simulink model "rx2"  (R2022b)
settings: Solver=FixedStepDiscrete  StartTime=0.0  StopTime=3.3E6  FixedStep=1  RelTol=1e-3  EnableMultiTasking=on
model workspace (MAT data in the model file):
  mwTaskManagerKernelLatency = 0
undefined symbols (not defined in the file or in its folder): Add, jsin, magnitude, rom_pilot_conj_tt, Shift
libraries: hdlsllib x3231, whdlutilities x525, simulink x260, whdlmod x112, whdledac x26, dsphdlmathfun2 x24, commchan3 x1
(part 42 of 59)

== system rx2/process3/decoder/p-p/Subsystem2/Subsystem1 ==
  data1 : Inport  OutDataTypeStr=data_type
  wr_addr : Inport  Port=2
  wr_en1 : Inport  Port=3
  rd_addr : Inport  Port=4
  Mux : Mux  Inputs=2
  Selector : Selector  InputPortWidth=32  IndexOptions=Index vector (dialog)  Indices=[1:16]  OutputSizes=1
  Selector1 : Selector  InputPortWidth=32  IndexOptions=Index vector (dialog)  Indices=[17:32]  OutputSizes=1
  Subsystem1 : Subsystem
  Subsystem2 : Subsystem
  rd_dout : Outport  PortDimensions=32  VectorParamsAs1DForOutWhenUnconnected=off
  wires:
  Selector1/1 -> Subsystem1/1(data1)
  Selector/1 -> Subsystem2/1(data1)
  rd_addr/1 -> Subsystem2/4(rd_addr), Subsystem1/4(rd_addr)
  Mux/1 -> rd_dout/1
  wr_en1/1 -> Subsystem2/3(wr_en1), Subsystem1/3(wr_en1)
  Subsystem2/1(rd_dout) -> Mux/1
  Subsystem1/1(rd_dout) -> Mux/2
  wr_addr/1 -> Subsystem2/2(wr_addr), Subsystem1/2(wr_addr)
  data1/1 -> Selector1/1, Selector/1

== system rx2/process3/decoder/p-p/p_s_new/Subsystem1 ==
  In1 : Inport
  Demux{,1..6} (7 alike) : Demux  Outputs=2
  Out1 : Outport
  Out2 : Outport  Port=2
  Out3 : Outport  Port=3
  Out4 : Outport  Port=4
  Out5 : Outport  Port=5
  Out6 : Outport  Port=6
  Out7 : Outport  Port=7
  Out8 : Outport  Port=8
  wires:
  Demux3/1 -> Out1/1
  Demux6/2 -> Out8/1
  Demux4/2 -> Out4/1
  Demux5/1 -> Out5/1
  In1/1 -> Demux2/1
  Demux5/2 -> Out6/1
  Demux3/2 -> Out2/1
  Demux1/1 -> Demux5/1
  Demux/2 -> Demux4/1
  Demux1/2 -> Demux6/1
  Demux6/1 -> Out7/1
  Demux2/2 -> Demux1/1
  Demux/1 -> Demux3/1
  Demux4/1 -> Out3/1
  Demux2/1 -> Demux/1

== system rx2/process3/decoder/p-p/p_s_new/Subsystem3 ==
  In1 : Inport
  Demux{,1..6} (7 alike) : Demux  Outputs=2
  Out1 : Outport
  Out2 : Outport  Port=2
  Out3 : Outport  Port=3
  Out4 : Outport  Port=4
  Out5 : Outport  Port=5
  Out6 : Outport  Port=6
  Out7 : Outport  Port=7
  Out8 : Outport  Port=8
  wires:
  Demux2/1 -> Demux/1
  Demux4/1 -> Out3/1
  Demux/1 -> Demux3/1
  Demux2/2 -> Demux1/1
  Demux6/1 -> Out7/1
  Demux1/2 -> Demux6/1
  Demux/2 -> Demux4/1
  Demux1/1 -> Demux5/1
  Demux3/2 -> Out2/1
  Demux5/2 -> Out6/1
  In1/1 -> Demux2/1
  Demux5/1 -> Out5/1
  Demux4/2 -> Out4/1
  Demux6/2 -> Out8/1
  Demux3/1 -> Out1/1

== system rx2/process3/decoder/p-p/p_s_new/Subsystem4 ==
  In1 : Inport
  Demux{,1..6} (7 alike) : Demux  Outputs=2
  Out1 : Outport
  Out2 : Outport  Port=2
  Out3 : Outport  Port=3
  Out4 : Outport  Port=4
  Out5 : Outport  Port=5
  Out6 : Outport  Port=6
  Out7 : Outport  Port=7
  Out8 : Outport  Port=8
  wires:
  Demux3/1 -> Out1/1
  Demux6/2 -> Out8/1
  Demux4/2 -> Out4/1
  Demux5/1 -> Out5/1
  In1/1 -> Demux2/1
  Demux5/2 -> Out6/1
  Demux3/2 -> Out2/1
  Demux1/1 -> Demux5/1
  Demux/2 -> Demux4/1
  Demux1/2 -> Demux6/1
  Demux6/1 -> Out7/1
  Demux2/2 -> Demux1/1
  Demux/1 -> Demux3/1
  Demux4/1 -> Out3/1
  Demux2/1 -> Demux/1

== system rx2/process3/decoder/p-p/p_s_new/Subsystem5 ==
  In1 : Inport
  Demux{,1..6} (7 alike) : Demux  Outputs=2
  Out1 : Outport
  Out2 : Outport  Port=2
  Out3 : Outport  Port=3
  Out4 : Outport  Port=4
  Out5 : Outport  Port=5
  Out6 : Outport  Port=6
  Out7 : Outport  Port=7
  Out8 : Outport  Port=8
  wires:
  Demux2/1 -> Demux/1
  Demux4/1 -> Out3/1
  Demux/1 -> Demux3/1
  Demux2/2 -> Demux1/1
  Demux6/1 -> Out7/1
  Demux1/2 -> Demux6/1
  Demux/2 -> Demux4/1
  Demux1/1 -> Demux5/1
  Demux3/2 -> Out2/1
  Demux5/2 -> Out6/1
  In1/1 -> Demux2/1
  Demux5/1 -> Out5/1
  Demux4/2 -> Out4/1
  Demux6/2 -> Out8/1
  Demux3/1 -> Out1/1

== system rx2/process4/decoder/p-p/Subsystem2/Subsystem ==
  data1 : Inport  OutDataTypeStr=data_type
  wr_addr : Inport  Port=2
  wr_en1 : Inport  Port=3
  rd_addr : Inport  Port=4
  Mux : Mux  Inputs=2
  Selector : Selector  InputPortWidth=32  IndexOptions=Index vector (dialog)  Indices=[1:16]  OutputSizes=1
  Selector1 : Selector  InputPortWidth=32  IndexOptions=Index vector (dialog)  Indices=[17:32]  OutputSizes=1
  Subsystem1 : Subsystem
  Subsystem2 : Subsystem
  rd_dout : Outport  PortDimensions=32  VectorParamsAs1DForOutWhenUnconnected=off
  wires:
  data1/1 -> Selector/1, Selector1/1
  wr_addr/1 -> Subsystem1/2(wr_addr), Subsystem2/2(wr_addr)
  Subsystem1/1(rd_dout) -> Mux/2
  Subsystem2/1(rd_dout) -> Mux/1
  wr_en1/1 -> Subsystem1/3(wr_en1), Subsystem2/3(wr_en1)
  Mux/1 -> rd_dout/1
  rd_addr/1 -> Subsystem1/4(rd_addr), Subsystem2/4(rd_addr)
  Selector/1 -> Subsystem2/1(data1)
  Selector1/1 -> Subsystem1/1(data1)

== system rx2/process4/decoder/p-p/Subsystem2/Subsystem1 ==
  data1 : Inport  OutDataTypeStr=data_type
  wr_addr : Inport  Port=2
  wr_en1 : Inport  Port=3
  rd_addr : Inport  Port=4
  Mux : Mux  Inputs=2
  Selector : Selector  InputPortWidth=32  IndexOptions=Index vector (dialog)  Indices=[1:16]  OutputSizes=1
  Selector1 : Selector  InputPortWidth=32  IndexOptions=Index vector (dialog)  Indices=[17:32]  OutputSizes=1
  Subsystem1 : Subsystem
  Subsystem2 : Subsystem
  rd_dout : Outport  PortDimensions=32  VectorParamsAs1DForOutWhenUnconnected=off
  wires:
  data1/1 -> Selector/1, Selector1/1
  wr_addr/1 -> Subsystem1/2(wr_addr), Subsystem2/2(wr_addr)
  Subsystem1/1(rd_dout) -> Mux/2
  Subsystem2/1(rd_dout) -> Mux/1
  wr_en1/1 -> Subsystem1/3(wr_en1), Subsystem2/3(wr_en1)
  Mux/1 -> rd_dout/1
  rd_addr/1 -> Subsystem1/4(rd_addr), Subsystem2/4(rd_addr)
  Selector/1 -> Subsystem2/1(data1)
  Selector1/1 -> Subsystem1/1(data1)

== system rx2/process4/decoder/p-p/p_s_new/Subsystem1 ==
  In1 : Inport
  Demux{,1..6} (7 alike) : Demux  Outputs=2
  Out1 : Outport
  Out2 : Outport  Port=2
  Out3 : Outport  Port=3
  Out4 : Outport  Port=4
  Out5 : Outport  Port=5
  Out6 : Outport  Port=6
  Out7 : Outport  Port=7
  Out8 : Outport  Port=8
  wires:
  Demux2/1 -> Demux/1
  Demux4/1 -> Out3/1
  Demux/1 -> Demux3/1
  Demux2/2 -> Demux1/1
  Demux6/1 -> Out7/1
  Demux1/2 -> Demux6/1
  Demux/2 -> Demux4/1
  Demux1/1 -> Demux5/1
  Demux3/2 -> Out2/1
  Demux5/2 -> Out6/1
  In1/1 -> Demux2/1
  Demux5/1 -> Out5/1
  Demux4/2 -> Out4/1
  Demux6/2 -> Out8/1
  Demux3/1 -> Out1/1

== system rx2/process4/decoder/p-p/p_s_new/Subsystem3 ==
  In1 : Inport
  Demux{,1..6} (7 alike) : Demux  Outputs=2
  Out1 : Outport
  Out2 : Outport  Port=2
  Out3 : Outport  Port=3
  Out4 : Outport  Port=4
  Out5 : Outport  Port=5
  Out6 : Outport  Port=6
  Out7 : Outport  Port=7
  Out8 : Outport  Port=8
  wires:
  Demux3/1 -> Out1/1
  Demux6/2 -> Out8/1
  Demux4/2 -> Out4/1
  Demux5/1 -> Out5/1
  In1/1 -> Demux2/1
  Demux5/2 -> Out6/1
  Demux3/2 -> Out2/1
  Demux1/1 -> Demux5/1
  Demux/2 -> Demux4/1
  Demux1/2 -> Demux6/1
  Demux6/1 -> Out7/1
  Demux2/2 -> Demux1/1
  Demux/1 -> Demux3/1
  Demux4/1 -> Out3/1
  Demux2/1 -> Demux/1

== system rx2/process4/decoder/p-p/p_s_new/Subsystem4 ==
  In1 : Inport
  Demux{,1..6} (7 alike) : Demux  Outputs=2
  Out1 : Outport
  Out2 : Outport  Port=2
  Out3 : Outport  Port=3
  Out4 : Outport  Port=4
  Out5 : Outport  Port=5
  Out6 : Outport  Port=6
  Out7 : Outport  Port=7
  Out8 : Outport  Port=8
  wires:
  Demux2/1 -> Demux/1
  Demux4/1 -> Out3/1
  Demux/1 -> Demux3/1
  Demux2/2 -> Demux1/1
  Demux6/1 -> Out7/1
  Demux1/2 -> Demux6/1
  Demux/2 -> Demux4/1
  Demux1/1 -> Demux5/1
  Demux3/2 -> Out2/1
  Demux5/2 -> Out6/1
  In1/1 -> Demux2/1
  Demux5/1 -> Out5/1
  Demux4/2 -> Out4/1
  Demux6/2 -> Out8/1
  Demux3/1 -> Out1/1

== system rx2/process4/decoder/p-p/p_s_new/Subsystem5 ==
  In1 : Inport
  Demux{,1..6} (7 alike) : Demux  Outputs=2
  Out1 : Outport
  Out2 : Outport  Port=2
  Out3 : Outport  Port=3
  Out4 : Outport  Port=4
  Out5 : Outport  Port=5
  Out6 : Outport  Port=6
  Out7 : Outport  Port=7
  Out8 : Outport  Port=8
  wires:
  Demux3/1 -> Out1/1
  Demux6/2 -> Out8/1
  Demux4/2 -> Out4/1
  Demux5/1 -> Out5/1
  In1/1 -> Demux2/1
  Demux5/2 -> Out6/1
  Demux3/2 -> Out2/1
  Demux1/1 -> Demux5/1
  Demux/2 -> Demux4/1
  Demux1/2 -> Demux6/1
  Demux6/1 -> Out7/1
  Demux2/2 -> Demux1/1
  Demux/1 -> Demux3/1
  Demux4/1 -> Out3/1
  Demux2/1 -> Demux/1

== system rx2/process5/decoder/p-p/Subsystem2/Subsystem ==
  data1 : Inport  OutDataTypeStr=data_type
  wr_addr : Inport  Port=2
  wr_en1 : Inport  Port=3
  rd_addr : Inport  Port=4
  Mux : Mux  Inputs=2
  Selector : Selector  InputPortWidth=32  IndexOptions=Index vector (dialog)  Indices=[1:16]  OutputSizes=1
  Selector1 : Selector  InputPortWidth=32  IndexOptions=Index vector (dialog)  Indices=[17:32]  OutputSizes=1
  Subsystem1 : Subsystem
  Subsystem2 : Subsystem
  rd_dout : Outport  PortDimensions=32  VectorParamsAs1DForOutWhenUnconnected=off
  wires:
  Selector1/1 -> Subsystem1/1(data1)
  Selector/1 -> Subsystem2/1(data1)
  rd_addr/1 -> Subsystem2/4(rd_addr), Subsystem1/4(rd_addr)
  Mux/1 -> rd_dout/1
  wr_en1/1 -> Subsystem2/3(wr_en1), Subsystem1/3(wr_en1)
  Subsystem2/1(rd_dout) -> Mux/1
  Subsystem1/1(rd_dout) -> Mux/2
  wr_addr/1 -> Subsystem2/2(wr_addr), Subsystem1/2(wr_addr)
  data1/1 -> Selector1/1, Selector/1

== system rx2/process5/decoder/p-p/Subsystem2/Subsystem1 ==
  data1 : Inport  OutDataTypeStr=data_type
  wr_addr : Inport  Port=2
  wr_en1 : Inport  Port=3
  rd_addr : Inport  Port=4
  Mux : Mux  Inputs=2
  Selector : Selector  InputPortWidth=32  IndexOptions=Index vector (dialog)  Indices=[1:16]  OutputSizes=1
  Selector1 : Selector  InputPortWidth=32  IndexOptions=Index vector (dialog)  Indices=[17:32]  OutputSizes=1
  Subsystem1 : Subsystem
  Subsystem2 : Subsystem
  rd_dout : Outport  PortDimensions=32  VectorParamsAs1DForOutWhenUnconnected=off
  wires:
  Selector1/1 -> Subsystem1/1(data1)
  Selector/1 -> Subsystem2/1(data1)
  rd_addr/1 -> Subsystem2/4(rd_addr), Subsystem1/4(rd_addr)
  Mux/1 -> rd_dout/1
  wr_en1/1 -> Subsystem2/3(wr_en1), Subsystem1/3(wr_en1)
  Subsystem2/1(rd_dout) -> Mux/1
  Subsystem1/1(rd_dout) -> Mux/2
  wr_addr/1 -> Subsystem2/2(wr_addr), Subsystem1/2(wr_addr)
  data1/1 -> Selector1/1, Selector/1

== system rx2/process5/decoder/p-p/p_s_new/Subsystem1 ==
  In1 : Inport
  Demux{,1..6} (7 alike) : Demux  Outputs=2
  Out1 : Outport
  Out2 : Outport  Port=2
  Out3 : Outport  Port=3
  Out4 : Outport  Port=4
  Out5 : Outport  Port=5
  Out6 : Outport  Port=6
  Out7 : Outport  Port=7
  Out8 : Outport  Port=8
  wires:
  Demux3/1 -> Out1/1
  Demux6/2 -> Out8/1
  Demux4/2 -> Out4/1
  Demux5/1 -> Out5/1
  In1/1 -> Demux2/1
  Demux5/2 -> Out6/1
  Demux3/2 -> Out2/1
  Demux1/1 -> Demux5/1
  Demux/2 -> Demux4/1
  Demux1/2 -> Demux6/1
  Demux6/1 -> Out7/1
  Demux2/2 -> Demux1/1
  Demux/1 -> Demux3/1
  Demux4/1 -> Out3/1
  Demux2/1 -> Demux/1

== system rx2/process5/decoder/p-p/p_s_new/Subsystem3 ==
  In1 : Inport
  Demux{,1..6} (7 alike) : Demux  Outputs=2
  Out1 : Outport
  Out2 : Outport  Port=2
  Out3 : Outport  Port=3
  Out4 : Outport  Port=4
  Out5 : Outport  Port=5
  Out6 : Outport  Port=6
  Out7 : Outport  Port=7
  Out8 : Outport  Port=8
  wires:
  Demux2/1 -> Demux/1
  Demux4/1 -> Out3/1
  Demux/1 -> Demux3/1
  Demux2/2 -> Demux1/1
  Demux6/1 -> Out7/1
  Demux1/2 -> Demux6/1
  Demux/2 -> Demux4/1
  Demux1/1 -> Demux5/1
  Demux3/2 -> Out2/1
  Demux5/2 -> Out6/1
  In1/1 -> Demux2/1
  Demux5/1 -> Out5/1
  Demux4/2 -> Out4/1
  Demux6/2 -> Out8/1
  Demux3/1 -> Out1/1

== system rx2/process5/decoder/p-p/p_s_new/Subsystem4 ==
  In1 : Inport
  Demux{,1..6} (7 alike) : Demux  Outputs=2
  Out1 : Outport
  Out2 : Outport  Port=2
  Out3 : Outport  Port=3
  Out4 : Outport  Port=4
  Out5 : Outport  Port=5
  Out6 : Outport  Port=6
  Out7 : Outport  Port=7
  Out8 : Outport  Port=8
  wires:
  Demux3/1 -> Out1/1
  Demux6/2 -> Out8/1
  Demux4/2 -> Out4/1
  Demux5/1 -> Out5/1
  In1/1 -> Demux2/1
  Demux5/2 -> Out6/1
  Demux3/2 -> Out2/1
  Demux1/1 -> Demux5/1
  Demux/2 -> Demux4/1
  Demux1/2 -> Demux6/1
  Demux6/1 -> Out7/1
  Demux2/2 -> Demux1/1
  Demux/1 -> Demux3/1
  Demux4/1 -> Out3/1
  Demux2/1 -> Demux/1

== system rx2/process5/decoder/p-p/p_s_new/Subsystem5 ==
  In1 : Inport
  Demux{,1..6} (7 alike) : Demux  Outputs=2
  Out1 : Outport
  Out2 : Outport  Port=2
  Out3 : Outport  Port=3
  Out4 : Outport  Port=4
  Out5 : Outport  Port=5
  Out6 : Outport  Port=6
  Out7 : Outport  Port=7
  Out8 : Outport  Port=8
  wires:
  Demux2/1 -> Demux/1
  Demux4/1 -> Out3/1
  Demux/1 -> Demux3/1
  Demux2/2 -> Demux1/1
  Demux6/1 -> Out7/1
  Demux1/2 -> Demux6/1
  Demux/2 -> Demux4/1
  Demux1/1 -> Demux5/1
  Demux3/2 -> Out2/1
  Demux5/2 -> Out6/1
  In1/1 -> Demux2/1
  Demux5/1 -> Out5/1
  Demux4/2 -> Out4/1
  Demux6/2 -> Out8/1
  Demux3/1 -> Out1/1

== system rx2/process6/decoder/p-p/Subsystem2/Subsystem ==
  data1 : Inport  OutDataTypeStr=data_type
  wr_addr : Inport  Port=2
  wr_en1 : Inport  Port=3
  rd_addr : Inport  Port=4
  Mux : Mux  Inputs=2
  Selector : Selector  InputPortWidth=32  IndexOptions=Index vector (dialog)  Indices=[1:16]  OutputSizes=1
  Selector1 : Selector  InputPortWidth=32  IndexOptions=Index vector (dialog)  Indices=[17:32]  OutputSizes=1
  Subsystem1 : Subsystem
  Subsystem2 : Subsystem
  rd_dout : Outport  PortDimensions=32  VectorParamsAs1DForOutWhenUnconnected=off
  wires:
  data1/1 -> Selector/1, Selector1/1
  wr_addr/1 -> Subsystem1/2(wr_addr), Subsystem2/2(wr_addr)
  Subsystem1/1(rd_dout) -> Mux/2
  Subsystem2/1(rd_dout) -> Mux/1
  wr_en1/1 -> Subsystem1/3(wr_en1), Subsystem2/3(wr_en1)
  Mux/1 -> rd_dout/1
  rd_addr/1 -> Subsystem1/4(rd_addr), Subsystem2/4(rd_addr)
  Selector/1 -> Subsystem2/1(data1)
  Selector1/1 -> Subsystem1/1(data1)

== system rx2/process6/decoder/p-p/Subsystem2/Subsystem1 ==
  data1 : Inport  OutDataTypeStr=data_type
  wr_addr : Inport  Port=2
  wr_en1 : Inport  Port=3
  rd_addr : Inport  Port=4
  Mux : Mux  Inputs=2
  Selector : Selector  InputPortWidth=32  IndexOptions=Index vector (dialog)  Indices=[1:16]  OutputSizes=1
  Selector1 : Selector  InputPortWidth=32  IndexOptions=Index vector (dialog)  Indices=[17:32]  OutputSizes=1
  Subsystem1 : Subsystem
  Subsystem2 : Subsystem
  rd_dout : Outport  PortDimensions=32  VectorParamsAs1DForOutWhenUnconnected=off
  wires:
  data1/1 -> Selector/1, Selector1/1
  wr_addr/1 -> Subsystem1/2(wr_addr), Subsystem2/2(wr_addr)
  Subsystem1/1(rd_dout) -> Mux/2
  Subsystem2/1(rd_dout) -> Mux/1
  wr_en1/1 -> Subsystem1/3(wr_en1), Subsystem2/3(wr_en1)
  Mux/1 -> rd_dout/1
  rd_addr/1 -> Subsystem1/4(rd_addr), Subsystem2/4(rd_addr)
  Selector/1 -> Subsystem2/1(data1)
  Selector1/1 -> Subsystem1/1(data1)

== system rx2/process6/decoder/p-p/p_s_new/Subsystem1 ==
  In1 : Inport
  Demux{,1..6} (7 alike) : Demux  Outputs=2
  Out1 : Outport
  Out2 : Outport  Port=2
  Out3 : Outport  Port=3
  Out4 : Outport  Port=4
  Out5 : Outport  Port=5
  Out6 : Outport  Port=6
  Out7 : Outport  Port=7
  Out8 : Outport  Port=8
  wires:
  Demux2/1 -> Demux/1
  Demux4/1 -> Out3/1
  Demux/1 -> Demux3/1
  Demux2/2 -> Demux1/1
  Demux6/1 -> Out7/1
  Demux1/2 -> Demux6/1
  Demux/2 -> Demux4/1
  Demux1/1 -> Demux5/1
  Demux3/2 -> Out2/1
  Demux5/2 -> Out6/1
  In1/1 -> Demux2/1
  Demux5/1 -> Out5/1
  Demux4/2 -> Out4/1
  Demux6/2 -> Out8/1
  Demux3/1 -> Out1/1

== system rx2/process6/decoder/p-p/p_s_new/Subsystem3 ==
  In1 : Inport
  Demux{,1..6} (7 alike) : Demux  Outputs=2
  Out1 : Outport
  Out2 : Outport  Port=2
  Out3 : Outport  Port=3
  Out4 : Outport  Port=4
  Out5 : Outport  Port=5
  Out6 : Outport  Port=6
  Out7 : Outport  Port=7
  Out8 : Outport  Port=8
  wires:
  Demux3/1 -> Out1/1
  Demux6/2 -> Out8/1
  Demux4/2 -> Out4/1
  Demux5/1 -> Out5/1
  In1/1 -> Demux2/1
  Demux5/2 -> Out6/1
  Demux3/2 -> Out2/1
  Demux1/1 -> Demux5/1
  Demux/2 -> Demux4/1
  Demux1/2 -> Demux6/1
  Demux6/1 -> Out7/1
  Demux2/2 -> Demux1/1
  Demux/1 -> Demux3/1
  Demux4/1 -> Out3/1
  Demux2/1 -> Demux/1

== system rx2/process6/decoder/p-p/p_s_new/Subsystem4 ==
  In1 : Inport
  Demux{,1..6} (7 alike) : Demux  Outputs=2
  Out1 : Outport
  Out2 : Outport  Port=2
  Out3 : Outport  Port=3
  Out4 : Outport  Port=4
  Out5 : Outport  Port=5
  Out6 : Outport  Port=6
  Out7 : Outport  Port=7
  Out8 : Outport  Port=8
  wires:
  Demux2/1 -> Demux/1
  Demux4/1 -> Out3/1
  Demux/1 -> Demux3/1
  Demux2/2 -> Demux1/1
  Demux6/1 -> Out7/1
  Demux1/2 -> Demux6/1
  Demux/2 -> Demux4/1
  Demux1/1 -> Demux5/1
  Demux3/2 -> Out2/1
  Demux5/2 -> Out6/1
  In1/1 -> Demux2/1
  Demux5/1 -> Out5/1
  Demux4/2 -> Out4/1
  Demux6/2 -> Out8/1
  Demux3/1 -> Out1/1

== system rx2/process6/decoder/p-p/p_s_new/Subsystem5 ==
  In1 : Inport
  Demux{,1..6} (7 alike) : Demux  Outputs=2
  Out1 : Outport
  Out2 : Outport  Port=2
  Out3 : Outport  Port=3
  Out4 : Outport  Port=4
  Out5 : Outport  Port=5
  Out6 : Outport  Port=6
  Out7 : Outport  Port=7
  Out8 : Outport  Port=8
  wires:
  Demux3/1 -> Out1/1
  Demux6/2 -> Out8/1
  Demux4/2 -> Out4/1
  Demux5/1 -> Out5/1
  In1/1 -> Demux2/1
  Demux5/2 -> Out6/1
  Demux3/2 -> Out2/1
  Demux1/1 -> Demux5/1
  Demux/2 -> Demux4/1
  Demux1/2 -> Demux6/1
  Demux6/1 -> Out7/1
  Demux2/2 -> Demux1/1
  Demux/1 -> Demux3/1
  Demux4/1 -> Out3/1
  Demux2/1 -> Demux/1

== system rx2/process7/decoder/p-p/Subsystem2/Subsystem ==
  data1 : Inport  OutDataTypeStr=data_type
  wr_addr : Inport  Port=2
  wr_en1 : Inport  Port=3
  rd_addr : Inport  Port=4
  Mux : Mux  Inputs=2
  Selector : Selector  InputPortWidth=32  IndexOptions=Index vector (dialog)  Indices=[1:16]  OutputSizes=1
  Selector1 : Selector  InputPortWidth=32  IndexOptions=Index vector (dialog)  Indices=[17:32]  OutputSizes=1
  Subsystem1 : Subsystem
  Subsystem2 : Subsystem
  rd_dout : Outport  PortDimensions=32  VectorParamsAs1DForOutWhenUnconnected=off
  wires:
  Selector1/1 -> Subsystem1/1(data1)
  Selector/1 -> Subsystem2/1(data1)
  rd_addr/1 -> Subsystem2/4(rd_addr), Subsystem1/4(rd_addr)
  Mux/1 -> rd_dout/1
  wr_en1/1 -> Subsystem2/3(wr_en1), Subsystem1/3(wr_en1)
  Subsystem2/1(rd_dout) -> Mux/1
  Subsystem1/1(rd_dout) -> Mux/2
  wr_addr/1 -> Subsystem2/2(wr_addr), Subsystem1/2(wr_addr)
  data1/1 -> Selector1/1, Selector/1

== system rx2/process7/decoder/p-p/Subsystem2/Subsystem1 ==
  data1 : Inport  OutDataTypeStr=data_type
  wr_addr : Inport  Port=2
  wr_en1 : Inport  Port=3
  rd_addr : Inport  Port=4
  Mux : Mux  Inputs=2
  Selector : Selector  InputPortWidth=32  IndexOptions=Index vector (dialog)  Indices=[1:16]  OutputSizes=1
  Selector1 : Selector  InputPortWidth=32  IndexOptions=Index vector (dialog)  Indices=[17:32]  OutputSizes=1
  Subsystem1 : Subsystem
  Subsystem2 : Subsystem
  rd_dout : Outport  PortDimensions=32  VectorParamsAs1DForOutWhenUnconnected=off
  wires:
  Selector1/1 -> Subsystem1/1(data1)
  Selector/1 -> Subsystem2/1(data1)
  rd_addr/1 -> Subsystem2/4(rd_addr), Subsystem1/4(rd_addr)
  Mux/1 -> rd_dout/1
  wr_en1/1 -> Subsystem2/3(wr_en1), Subsystem1/3(wr_en1)
  Subsystem2/1(rd_dout) -> Mux/1
  Subsystem1/1(rd_dout) -> Mux/2
  wr_addr/1 -> Subsystem2/2(wr_addr), Subsystem1/2(wr_addr)
  data1/1 -> Selector1/1, Selector/1

== system rx2/process7/decoder/p-p/p_s_new/Subsystem1 ==
  In1 : Inport
  Demux{,1..6} (7 alike) : Demux  Outputs=2
  Out1 : Outport
  Out2 : Outport  Port=2
  Out3 : Outport  Port=3
  Out4 : Outport  Port=4
  Out5 : Outport  Port=5
  Out6 : Outport  Port=6
  Out7 : Outport  Port=7
  Out8 : Outport  Port=8
  wires:
  Demux3/1 -> Out1/1
  Demux6/2 -> Out8/1
  Demux4/2 -> Out4/1
  Demux5/1 -> Out5/1
  In1/1 -> Demux2/1
  Demux5/2 -> Out6/1
  Demux3/2 -> Out2/1
  Demux1/1 -> Demux5/1
  Demux/2 -> Demux4/1
  Demux1/2 -> Demux6/1
  Demux6/1 -> Out7/1
  Demux2/2 -> Demux1/1
  Demux/1 -> Demux3/1
  Demux4/1 -> Out3/1
  Demux2/1 -> Demux/1

== system rx2/process7/decoder/p-p/p_s_new/Subsystem3 ==
  In1 : Inport
  Demux{,1..6} (7 alike) : Demux  Outputs=2
  Out1 : Outport
  Out2 : Outport  Port=2
  Out3 : Outport  Port=3
  Out4 : Outport  Port=4
  Out5 : Outport  Port=5
  Out6 : Outport  Port=6
  Out7 : Outport  Port=7
  Out8 : Outport  Port=8
  wires:
  Demux2/1 -> Demux/1
  Demux4/1 -> Out3/1
  Demux/1 -> Demux3/1
  Demux2/2 -> Demux1/1
  Demux6/1 -> Out7/1
  Demux1/2 -> Demux6/1
  Demux/2 -> Demux4/1
  Demux1/1 -> Demux5/1
  Demux3/2 -> Out2/1
  Demux5/2 -> Out6/1
  In1/1 -> Demux2/1
  Demux5/1 -> Out5/1
  Demux4/2 -> Out4/1
  Demux6/2 -> Out8/1
  Demux3/1 -> Out1/1

== system rx2/process7/decoder/p-p/p_s_new/Subsystem4 ==
  In1 : Inport
  Demux{,1..6} (7 alike) : Demux  Outputs=2
  Out1 : Outport
  Out2 : Outport  Port=2
  Out3 : Outport  Port=3
  Out4 : Outport  Port=4
  Out5 : Outport  Port=5
  Out6 : Outport  Port=6
  Out7 : Outport  Port=7
  Out8 : Outport  Port=8
  wires:
  Demux3/1 -> Out1/1
  Demux6/2 -> Out8/1
  Demux4/2 -> Out4/1
  Demux5/1 -> Out5/1
  In1/1 -> Demux2/1
  Demux5/2 -> Out6/1
  Demux3/2 -> Out2/1
  Demux1/1 -> Demux5/1
  Demux/2 -> Demux4/1
  Demux1/2 -> Demux6/1
  Demux6/1 -> Out7/1
  Demux2/2 -> Demux1/1
  Demux/1 -> Demux3/1
  Demux4/1 -> Out3/1
  Demux2/1 -> Demux/1

== system rx2/process7/decoder/p-p/p_s_new/Subsystem5 ==
  In1 : Inport
  Demux{,1..6} (7 alike) : Demux  Outputs=2
  Out1 : Outport
  Out2 : Outport  Port=2
  Out3 : Outport  Port=3
  Out4 : Outport  Port=4
  Out5 : Outport  Port=5
  Out6 : Outport  Port=6
  Out7 : Outport  Port=7
  Out8 : Outport  Port=8
  wires:
  Demux2/1 -> Demux/1
  Demux4/1 -> Out3/1
  Demux/1 -> Demux3/1
  Demux2/2 -> Demux1/1
  Demux6/1 -> Out7/1
  Demux1/2 -> Demux6/1
  Demux/2 -> Demux4/1
  Demux1/1 -> Demux5/1
  Demux3/2 -> Out2/1
  Demux5/2 -> Out6/1
  In1/1 -> Demux2/1
  Demux5/1 -> Out5/1
  Demux4/2 -> Out4/1
  Demux6/2 -> Out8/1
  Demux3/1 -> Out1/1

== system rx2/process8/decoder/p-p/Subsystem2/Subsystem ==
  data1 : Inport  OutDataTypeStr=data_type
  wr_addr : Inport  Port=2
  wr_en1 : Inport  Port=3
  rd_addr : Inport  Port=4
  Mux : Mux  Inputs=2
  Selector : Selector  InputPortWidth=32  IndexOptions=Index vector (dialog)  Indices=[1:16]  OutputSizes=1
  Selector1 : Selector  InputPortWidth=32  IndexOptions=Index vector (dialog)  Indices=[17:32]  OutputSizes=1
  Subsystem1 : Subsystem
  Subsystem2 : Subsystem
  rd_dout : Outport  PortDimensions=32  VectorParamsAs1DForOutWhenUnconnected=off
  wires:
  data1/1 -> Selector/1, Selector1/1
  wr_addr/1 -> Subsystem1/2(wr_addr), Subsystem2/2(wr_addr)
  Subsystem1/1(rd_dout) -> Mux/2
  Subsystem2/1(rd_dout) -> Mux/1
  wr_en1/1 -> Subsystem1/3(wr_en1), Subsystem2/3(wr_en1)
  Mux/1 -> rd_dout/1
  rd_addr/1 -> Subsystem1/4(rd_addr), Subsystem2/4(rd_addr)
  Selector/1 -> Subsystem2/1(data1)
  Selector1/1 -> Subsystem1/1(data1)

== system rx2/process8/decoder/p-p/Subsystem2/Subsystem1 ==
  data1 : Inport  OutDataTypeStr=data_type
  wr_addr : Inport  Port=2
  wr_en1 : Inport  Port=3
  rd_addr : Inport  Port=4
  Mux : Mux  Inputs=2
  Selector : Selector  InputPortWidth=32  IndexOptions=Index vector (dialog)  Indices=[1:16]  OutputSizes=1
  Selector1 : Selector  InputPortWidth=32  IndexOptions=Index vector (dialog)  Indices=[17:32]  OutputSizes=1
  Subsystem1 : Subsystem
  Subsystem2 : Subsystem
  rd_dout : Outport  PortDimensions=32  VectorParamsAs1DForOutWhenUnconnected=off
  wires:
  data1/1 -> Selector/1, Selector1/1
  wr_addr/1 -> Subsystem1/2(wr_addr), Subsystem2/2(wr_addr)
  Subsystem1/1(rd_dout) -> Mux/2
  Subsystem2/1(rd_dout) -> Mux/1
  wr_en1/1 -> Subsystem1/3(wr_en1), Subsystem2/3(wr_en1)
  Mux/1 -> rd_dout/1
  rd_addr/1 -> Subsystem1/4(rd_addr), Subsystem2/4(rd_addr)
  Selector/1 -> Subsystem2/1(data1)
  Selector1/1 -> Subsystem1/1(data1)

== system rx2/process8/decoder/p-p/p_s_new/Subsystem1 ==
  In1 : Inport
  Demux{,1..6} (7 alike) : Demux  Outputs=2
  Out1 : Outport
  Out2 : Outport  Port=2
  Out3 : Outport  Port=3
  Out4 : Outport  Port=4
  Out5 : Outport  Port=5
  Out6 : Outport  Port=6
  Out7 : Outport  Port=7
  Out8 : Outport  Port=8
  wires:
  Demux2/1 -> Demux/1
  Demux4/1 -> Out3/1
  Demux/1 -> Demux3/1
  Demux2/2 -> Demux1/1
  Demux6/1 -> Out7/1
  Demux1/2 -> Demux6/1
  Demux/2 -> Demux4/1
  Demux1/1 -> Demux5/1
  Demux3/2 -> Out2/1
  Demux5/2 -> Out6/1
  In1/1 -> Demux2/1
  Demux5/1 -> Out5/1
  Demux4/2 -> Out4/1
  Demux6/2 -> Out8/1
  Demux3/1 -> Out1/1

== system rx2/process8/decoder/p-p/p_s_new/Subsystem3 ==
  In1 : Inport
  Demux{,1..6} (7 alike) : Demux  Outputs=2
  Out1 : Outport
  Out2 : Outport  Port=2
  Out3 : Outport  Port=3
  Out4 : Outport  Port=4
  Out5 : Outport  Port=5
  Out6 : Outport  Port=6
  Out7 : Outport  Port=7
  Out8 : Outport  Port=8
  wires:
  Demux3/1 -> Out1/1
  Demux6/2 -> Out8/1
  Demux4/2 -> Out4/1
  Demux5/1 -> Out5/1
  In1/1 -> Demux2/1
  Demux5/2 -> Out6/1
  Demux3/2 -> Out2/1
  Demux1/1 -> Demux5/1
  Demux/2 -> Demux4/1
  Demux1/2 -> Demux6/1
  Demux6/1 -> Out7/1
  Demux2/2 -> Demux1/1
  Demux/1 -> Demux3/1
  Demux4/1 -> Out3/1
  Demux2/1 -> Demux/1

== system rx2/process8/decoder/p-p/p_s_new/Subsystem4 ==
  In1 : Inport
  Demux{,1..6} (7 alike) : Demux  Outputs=2
  Out1 : Outport
  Out2 : Outport  Port=2
  Out3 : Outport  Port=3
  Out4 : Outport  Port=4
  Out5 : Outport  Port=5
  Out6 : Outport  Port=6
  Out7 : Outport  Port=7
  Out8 : Outport  Port=8
  wires:
  Demux2/1 -> Demux/1
  Demux4/1 -> Out3/1
  Demux/1 -> Demux3/1
  Demux2/2 -> Demux1/1
  Demux6/1 -> Out7/1
  Demux1/2 -> Demux6/1
  Demux/2 -> Demux4/1
  Demux1/1 -> Demux5/1
  Demux3/2 -> Out2/1
  Demux5/2 -> Out6/1
  In1/1 -> Demux2/1
  Demux5/1 -> Out5/1
  Demux4/2 -> Out4/1
  Demux6/2 -> Out8/1
  Demux3/1 -> Out1/1

== system rx2/process8/decoder/p-p/p_s_new/Subsystem5 ==
  In1 : Inport
  Demux{,1..6} (7 alike) : Demux  Outputs=2
  Out1 : Outport
  Out2 : Outport  Port=2
  Out3 : Outport  Port=3
  Out4 : Outport  Port=4
  Out5 : Outport  Port=5
  Out6 : Outport  Port=6
  Out7 : Outport  Port=7
  Out8 : Outport  Port=8
  wires:
  Demux3/1 -> Out1/1
  Demux6/2 -> Out8/1
  Demux4/2 -> Out4/1
  Demux5/1 -> Out5/1
  In1/1 -> Demux2/1
  Demux5/2 -> Out6/1
  Demux3/2 -> Out2/1
  Demux1/1 -> Demux5/1
  Demux/2 -> Demux4/1
  Demux1/2 -> Demux6/1
  Demux6/1 -> Out7/1
  Demux2/2 -> Demux1/1
  Demux/1 -> Demux3/1
  Demux4/1 -> Out3/1
  Demux2/1 -> Demux/1

== system rx2/process9/decoder/p-p/Subsystem2/Subsystem ==
  data1 : Inport  OutDataTypeStr=data_type
  wr_addr : Inport  Port=2
  wr_en1 : Inport  Port=3
  rd_addr : Inport  Port=4
  Mux : Mux  Inputs=2
  Selector : Selector  InputPortWidth=32  IndexOptions=Index vector (dialog)  Indices=[1:16]  OutputSizes=1
  Selector1 : Selector  InputPortWidth=32  IndexOptions=Index vector (dialog)  Indices=[17:32]  OutputSizes=1
  Subsystem1 : Subsystem
  Subsystem2 : Subsystem
  rd_dout : Outport  PortDimensions=32  VectorParamsAs1DForOutWhenUnconnected=off
  wires:
  Selector1/1 -> Subsystem1/1(data1)
  Selector/1 -> Subsystem2/1(data1)
  rd_addr/1 -> Subsystem2/4(rd_addr), Subsystem1/4(rd_addr)
  Mux/1 -> rd_dout/1
  wr_en1/1 -> Subsystem2/3(wr_en1), Subsystem1/3(wr_en1)
  Subsystem2/1(rd_dout) -> Mux/1
  Subsystem1/1(rd_dout) -> Mux/2
  wr_addr/1 -> Subsystem2/2(wr_addr), Subsystem1/2(wr_addr)
  data1/1 -> Selector1/1, Selector/1

== system rx2/process9/decoder/p-p/Subsystem2/Subsystem1 ==
  data1 : Inport  OutDataTypeStr=data_type
  wr_addr : Inport  Port=2
  wr_en1 : Inport  Port=3
  rd_addr : Inport  Port=4
  Mux : Mux  Inputs=2
  Selector : Selector  InputPortWidth=32  IndexOptions=Index vector (dialog)  Indices=[1:16]  OutputSizes=1
  Selector1 : Selector  InputPortWidth=32  IndexOptions=Index vector (dialog)  Indices=[17:32]  OutputSizes=1
  Subsystem1 : Subsystem
  Subsystem2 : Subsystem
  rd_dout : Outport  PortDimensions=32  VectorParamsAs1DForOutWhenUnconnected=off
  wires:
  Selector1/1 -> Subsystem1/1(data1)
  Selector/1 -> Subsystem2/1(data1)
  rd_addr/1 -> Subsystem2/4(rd_addr), Subsystem1/4(rd_addr)
  Mux/1 -> rd_dout/1
  wr_en1/1 -> Subsystem2/3(wr_en1), Subsystem1/3(wr_en1)
  Subsystem2/1(rd_dout) -> Mux/1
  Subsystem1/1(rd_dout) -> Mux/2
  wr_addr/1 -> Subsystem2/2(wr_addr), Subsystem1/2(wr_addr)
  data1/1 -> Selector1/1, Selector/1

== system rx2/process9/decoder/p-p/p_s_new/Subsystem1 ==
  In1 : Inport
  Demux{,1..6} (7 alike) : Demux  Outputs=2
  Out1 : Outport
  Out2 : Outport  Port=2
  Out3 : Outport  Port=3
  Out4 : Outport  Port=4
  Out5 : Outport  Port=5
  Out6 : Outport  Port=6
  Out7 : Outport  Port=7
  Out8 : Outport  Port=8
  wires:
  Demux3/1 -> Out1/1
  Demux6/2 -> Out8/1
  Demux4/2 -> Out4/1
  Demux5/1 -> Out5/1
  In1/1 -> Demux2/1
  Demux5/2 -> Out6/1
  Demux3/2 -> Out2/1
  Demux1/1 -> Demux5/1
  Demux/2 -> Demux4/1
  Demux1/2 -> Demux6/1
  Demux6/1 -> Out7/1
  Demux2/2 -> Demux1/1
  Demux/1 -> Demux3/1
  Demux4/1 -> Out3/1
  Demux2/1 -> Demux/1

== system rx2/process9/decoder/p-p/p_s_new/Subsystem3 ==
  In1 : Inport
  Demux{,1..6} (7 alike) : Demux  Outputs=2
  Out1 : Outport
  Out2 : Outport  Port=2
  Out3 : Outport  Port=3
  Out4 : Outport  Port=4
  Out5 : Outport  Port=5
  Out6 : Outport  Port=6
  Out7 : Outport  Port=7
  Out8 : Outport  Port=8
  wires:
  Demux2/1 -> Demux/1
  Demux4/1 -> Out3/1
  Demux/1 -> Demux3/1
  Demux2/2 -> Demux1/1
  Demux6/1 -> Out7/1
  Demux1/2 -> Demux6/1
  Demux/2 -> Demux4/1
  Demux1/1 -> Demux5/1
  Demux3/2 -> Out2/1
  Demux5/2 -> Out6/1
  In1/1 -> Demux2/1
  Demux5/1 -> Out5/1
  Demux4/2 -> Out4/1
  Demux6/2 -> Out8/1
  Demux3/1 -> Out1/1

== system rx2/process9/decoder/p-p/p_s_new/Subsystem4 ==
  In1 : Inport
  Demux{,1..6} (7 alike) : Demux  Outputs=2
  Out1 : Outport
  Out2 : Outport  Port=2
  Out3 : Outport  Port=3
  Out4 : Outport  Port=4
  Out5 : Outport  Port=5
  Out6 : Outport  Port=6
  Out7 : Outport  Port=7
  Out8 : Outport  Port=8
  wires:
  Demux3/1 -> Out1/1
  Demux6/2 -> Out8/1
  Demux4/2 -> Out4/1
  Demux5/1 -> Out5/1
  In1/1 -> Demux2/1
  Demux5/2 -> Out6/1
  Demux3/2 -> Out2/1
  Demux1/1 -> Demux5/1
  Demux/2 -> Demux4/1
  Demux1/2 -> Demux6/1
  Demux6/1 -> Out7/1
  Demux2/2 -> Demux1/1
  Demux/1 -> Demux3/1
  Demux4/1 -> Out3/1
  Demux2/1 -> Demux/1

== system rx2/process9/decoder/p-p/p_s_new/Subsystem5 ==
  In1 : Inport
  Demux{,1..6} (7 alike) : Demux  Outputs=2
  Out1 : Outport
  Out2 : Outport  Port=2
  Out3 : Outport  Port=3
  Out4 : Outport  Port=4
  Out5 : Outport  Port=5
  Out6 : Outport  Port=6
  Out7 : Outport  Port=7
  Out8 : Outport  Port=8
  wires:
  Demux2/1 -> Demux/1
  Demux4/1 -> Out3/1
  Demux/1 -> Demux3/1
  Demux2/2 -> Demux1/1
  Demux6/1 -> Out7/1
  Demux1/2 -> Demux6/1
  Demux/2 -> Demux4/1
  Demux1/1 -> Demux5/1
  Demux3/2 -> Out2/1
  Demux5/2 -> Out6/1
  In1/1 -> Demux2/1
  Demux5/1 -> Out5/1
  Demux4/2 -> Out4/1
  Demux6/2 -> Out8/1
  Demux3/1 -> Out1/1

== system rx2/demode1/chan_est1/Subsystem/HDL_DUT/H_est/hRAM1 ==
  H_out : Inport  OutDataTypeStr=fixdt(1,32,27)  PortDimensions=1
  H_valid_out : Inport  Port=2  OutDataTypeStr=boolean
  H_end_out : Inport  Port=3  OutDataTypeStr=boolean
  Compare To Constant : hdlsllib/Logic and Bit Operations/Compare To Constant  relop===  const=10.0  OutDataTypeStr=boolean
  Constant : Constant  OutDataTypeStr=fixdt(0,2,0)
  Constant1 : Constant  OutDataTypeStr=fixdt(0,2,0)
  HDL Counter2 : hdlsllib/Sources/HDL Counter  CountType=Count limited  CountInit=0  CountStep=1  CountMax=11  CountFromType=Initial value  CountFrom=0  CountResetPort=on  CountLoadPort=off  CountEnbPort=on  CountDirPort=off  CountHitOutputPort=off  CountDataType=Unsigned  CountWordLen=8  CountFracLen=0  CountSampTime=1
  Simple Dual Port RAM : hdlsllib/HDL RAMs/Simple Dual Port RAM  ram_size=2
  Out1 : Outport  VectorParamsAs1DForOutWhenUnconnected=off
  wires:
  Compare To Constant/1 -> Simple Dual Port RAM/3
  H_out/1 -> Simple Dual Port RAM/1
  H_valid_out/1 -> HDL Counter2/2
  Constant/1 -> Simple Dual Port RAM/2
  HDL Counter2/1 -> Compare To Constant/1
  Simple Dual Port RAM/1 -> Out1/1
  Constant1/1 -> Simple Dual Port RAM/4
  H_end_out/1 -> HDL Counter2/1

== system rx2/demode1/chan_est1/Subsystem/HDL_DUT/LS_Est/ctrl_gen ==
  data_in : Inport
  valid_in : Inport  Port=2
  Delay : Delay  DelayLength=1  InitialCondition=0
  Delay1 : Delay  DelayLength=1  InitialCondition=0
  Delay2 : Delay  DelayLength=1  InitialCondition=0
  Detect Fall Nonpositive : hdlsllib/Logic and Bit Operations/Detect Fall Nonpositive  vinit=0  OutDataTypeStr=boolean
  Detect Rise Positive : hdlsllib/Logic and Bit Operations/Detect Rise Positive  vinit=0  OutDataTypeStr=boolean
  Sample Control Bus Creator : whdlutilities/Sample Control Bus Creator
  data_out : Outport
  ctrl_out : Outport  Port=2
  wires:
  Delay2/1 -> data_out/1
  data_in/1 -> Delay2/1
  Delay1/1 -> Detect Rise Positive/1
  Delay/1 -> Sample Control Bus Creator/3
  Sample Control Bus Creator/1 -> ctrl_out/1
  valid_in/1 -> Delay1/1, Detect Fall Nonpositive/1, Delay/1
  Detect Rise Positive/1 -> Sample Control Bus Creator/1
  Detect Fall Nonpositive/1 -> Sample Control Bus Creator/2

== system rx2/demode1/chan_est1/Subsystem/HDL_DUT/LS_Est/ctrl_gen1 ==
  valid_in : Inport
  Constant : Constant  Value=0
  Data Type Conversion : DataTypeConversion  OutDataTypeStr=boolean  SaturateOnIntegerOverflow=off  RndMeth=Floor
  HDL Counter1 : hdlsllib/Sources/HDL Counter  CountType=Count limited  CountInit=0  CountStep=1  CountMax=1024  CountFromType=Initial value  CountFrom=0  CountResetPort=on  CountLoadPort=off  CountEnbPort=on  CountDirPort=off  CountHitOutputPort=off  CountDataType=Unsigned  CountWordLen=16  CountFracLen=0  CountSampTime=1
  HDL Counter2 : hdlsllib/Sources/HDL Counter  CountType=Count limited  CountInit=0  CountStep=1  CountMax=1  CountFromType=Initial value  CountFrom=0  CountResetPort=off  CountLoadPort=off  CountEnbPort=on  CountDirPort=off  CountHitOutputPort=off  CountDataType=Unsigned  CountWordLen=16  CountFracLen=0  CountSampTime=1
  Logical Operator : Logic  Operator=NOT  AllPortsSameDT=off  OutDataTypeStr=boolean
  Switch : Switch  Threshold=792  OutDataTypeStr=boolean  SaturateOnIntegerOverflow=off  InputSameDT=off
  wvalid_out : Outport  VectorParamsAs1DForOutWhenUnconnected=off
  wires:
  valid_in/1 -> Switch/3, Logical Operator/1, HDL Counter1/2
  Logical Operator/1 -> HDL Counter1/1
  HDL Counter2/1 -> Data Type Conversion/1
  HDL Counter1/1 -> Switch/2
  Constant/1 -> Switch/1
  Switch/1 -> HDL Counter2/1
  Data Type Conversion/1 -> wvalid_out/1

== system rx2/demode1/chan_est1/Subsystem/HDL_DUT/Pliot/rom ==
  note: rom_pilot = [1+1j;0+0j;-1+1j;0+0j;-1-1j;0+0j;1-1j;0+0j]*1/sqrt(2);
      | rom_pilot_conj = conj(rom_pilot);
      | rom_pilot_conj_tt = fi(rom_pilot_conj,1,16,14);
  note: HDL ROM
  address : Inport
  Direct Lookup Table (n-D) : LookupNDDirect  NumberOfTableDimensions=1  Table=rom_pilot_conj_tt  DiagnosticForOutOfRangeInput=Error
  InputReg : Delay  DelayLength=1
  ResetNoneDelay : Delay  DelayLength=1
  data_out : Outport
  wires:
  ResetNoneDelay/1 -> data_out/1
  address/1 -> InputReg/1
  Direct Lookup Table (n-D)/1 -> ResetNoneDelay/1
  InputReg/1 -> Direct Lookup Table (n-D)/1  "rom_add"

== system rx2/demode1/chan_est1/Subsystem/HDL_DUT/TA_EST/ctrl_gen ==
  data_in : Inport
      settings: SignalType=complex
  valid_in : Inport  Port=2
  Delay : Delay  DelayLength=1  InitialCondition=0
  Delay1 : Delay  DelayLength=1  InitialCondition=0
  Delay2 : Delay  DelayLength=1  InitialCondition=0
  Detect Fall Nonpositive : hdlsllib/Logic and Bit Operations/Detect Fall Nonpositive  vinit=0  OutDataTypeStr=boolean
  Detect Rise Positive : hdlsllib/Logic and Bit Operations/Detect Rise Positive  vinit=0  OutDataTypeStr=boolean
  Sample Control Bus Creator : whdlutilities/Sample Control Bus Creator
  data_out : Outport
  ctrl_out : Outport  Port=2
  wires:
  Delay2/1 -> data_out/1
  data_in/1 -> Delay2/1
  Delay1/1 -> Detect Rise Positive/1
  Delay/1 -> Sample Control Bus Creator/3
  Sample Control Bus Creator/1 -> ctrl_out/1
  valid_in/1 -> Delay1/1, Detect Fall Nonpositive/1, Delay/1
  Detect Rise Positive/1 -> Sample Control Bus Creator/1
  Detect Fall Nonpositive/1 -> Sample Control Bus Creator/2

== system rx2/demode1/chan_est1/Subsystem/HDL_DUT/delta_estimator/calculate_norm2 ==
  data_in : Inport
  Complex to Real-Imag2 : ComplexToRealImag
  Dot Product2 : DotProduct  OutDataTypeStr=fixdt(1,64,56)
  Terminator : Terminator
  data_out : Outport
  wires:
  Complex to Real-Imag2/2 -> Terminator/1
  Complex to Real-Imag2/1 -> data_out/1
  data_in/1 -> Dot Product2/1, Dot Product2/2
  Dot Product2/1 -> Complex to Real-Imag2/1

== system rx2/demode1/chan_est1/Subsystem/HDL_DUT/delta_estimator/calculate_norm3 ==
  data_in : Inport
  Complex to Real-Imag2 : ComplexToRealImag
  Dot Product2 : DotProduct  OutDataTypeStr=fixdt(1,64,56)
  Terminator : Terminator
  data_out : Outport
  wires:
  Dot Product2/1 -> Complex to Real-Imag2/1
  data_in/1 -> Dot Product2/2, Dot Product2/1
  Complex to Real-Imag2/1 -> data_out/1
  Complex to Real-Imag2/2 -> Terminator/1

== system rx2/demode1/chan_est1/Subsystem/HDL_DUT/delta_estimator/iteration_estimation ==
  data_in : Inport  OutDataTypeStr=fixdt(1,17,14)
  valid_in : Inport  Port=2  OutDataTypeStr=boolean
  Add : Sum  Inputs=+-  OutDataTypeStr=fixdt(1,16,14)
  Add1 : Sum  AccumDataTypeStr=fixdt(1,32,28)  OutDataTypeStr=fixdt(1,32,28)
  Compare To Constant : hdlsllib/Logic and Bit Operations/Compare To Constant  relop===  const=1  OutDataTypeStr=boolean
  Delay : Delay  DelayLength=1  InitialCondition=0
  Delay1 : Delay  DelayLength=1  InitialCondition=0
  Delay2 : Delay  DelayLength=1  InitialCondition=0
  Ground : Ground
  HDL Counter : hdlsllib/Sources/HDL Counter  CountType=Count limited  CountInit=0  CountStep=1  CountMax=396  CountFromType=Initial value  CountFrom=0  CountResetPort=on  CountLoadPort=off  CountEnbPort=on  CountDirPort=off  CountHitOutputPort=on  CountDataType=Unsigned  CountWordLen=10  CountFracLen=0  CountSampTime=1
  Logical Operator : Logic  AllPortsSameDT=off  OutDataTypeStr=boolean
  Math Function : Math  Operator=reciprocal  SignedPower=on  OutDataTypeStr=fixdt(1,16,14)  RndMeth=Zero
  Product : Product
  Switch1 : Switch  Criteria=u2 ~= 0  SaturateOnIntegerOverflow=off  InputSameDT=off
  register : Subsystem
      settings: PortSchema="{\"entries\":[{\"content\":{\"sides\":[{\"content\":{\"connectorIds\":[\"In1\"]},\"type\":\"ConnectorPlacement.EquallySpacedRectSide\",\"uuid\":\"d2805390-6fde-484c-9a7d-6394e985dbe8\"},{\"content\":{\"connectorIds\":[\"Out1\"],\"side\":\"RIGHT\"},\"type\":\"ConnectorPlacement.EquallySpacedRectSide\",\"uuid\":\"b8bae0ca-bbac-4755-ad66-12c0db47e001\"},{\"content\":{\"connectorIds\":[],\"side\":\"TOP\"},\"type\":\"ConnectorPlacement.EquallySpacedRectSide\",\"uuid\":\"3b6f7ac7-ceca-420c-88f8-6d8200a607a4\"},{\"content\":{\"connectorIds\":[\"In2\",\"In3\"],\"side\":\"BOTTOM\"},\"type\":\"ConnectorPlacement.EquallySpacedRectSide\",\"uuid\":\"616043b2-e095-45f8-84b4-1e3ef3d522d8\"}]},\"type\":\"ConnectorPlacement.EquallySpacedConnector\",\"uuid\":\"94d0aeb7-2bda-42be-943a-50da35b391e1\"}],\"packageUris\":[\"http://schema.mathworks.com/mf0/Connector/R2020b\"],\"version\":\"1.0\"}"
  data_out : Outport  VectorParamsAs1DForOutWhenUnconnected=off
  valid_out : Outport  Port=2  OutDataTypeStr=boolean  VectorParamsAs1DForOutWhenUnconnected=off
  wires:
  Add/1 -> Product/1
  data_in/1 -> Delay/1
  register/1(data_out) -> Add/2, Add1/2
  Product/1 -> Add1/1
  Add1/1 -> register/1(data_in), Switch1/1  "out"
  valid_in/1 -> HDL Counter/2, Logical Operator/2, Delay2/1
  Math Function/1 -> Product/2
  Compare To Constant/1 -> Logical Operator/1
  Delay1/1 -> HDL Counter/1
  HDL Counter/1 -> Compare To Constant/1, Math Function/1
  HDL Counter/2 -> Delay1/1
  Logical Operator/1 -> register/3(to_0)
  Switch1/1 -> data_out/1
  Ground/1 -> Switch1/3
  Delay/1 -> Add/1
  Delay2/1 -> Switch1/2, valid_out/1, register/2(valid_in)

== system rx2/demode1/chan_est1/Subsystem/HDL_DUT/delta_estimator/iteration_estimation1 ==
  data_in : Inport  OutDataTypeStr=fixdt(1,32,28)
  valid_in : Inport  Port=2  OutDataTypeStr=boolean
  Add : Sum  Inputs=+-  OutDataTypeStr=fixdt(1,32,28)
  Add1 : Sum  AccumDataTypeStr=fixdt(1,32,28)  OutDataTypeStr=fixdt(1,32,28)
  Compare To Constant : hdlsllib/Logic and Bit Operations/Compare To Constant  relop===  const=1  OutDataTypeStr=boolean
  Compare To Constant1 : hdlsllib/Logic and Bit Operations/Compare To Constant  relop===  const=0  OutDataTypeStr=boolean
  Delay : Delay  DelayLength=1  InitialCondition=0
  Delay1 : Delay  DelayLength=1  InitialCondition=0
  Delay2 : Delay  DelayLength=1  InitialCondition=0
  From : From
  Goto : Goto
  Ground : Ground
  HDL Counter : hdlsllib/Sources/HDL Counter  CountType=Count limited  CountInit=0  CountStep=1  CountMax=396  CountFromType=Initial value  CountFrom=0  CountResetPort=on  CountLoadPort=off  CountEnbPort=on  CountDirPort=off  CountHitOutputPort=on  CountDataType=Unsigned  CountWordLen=10  CountFracLen=0  CountSampTime=1
  Logical Operator : Logic  AllPortsSameDT=off  OutDataTypeStr=boolean
  Math Function : Math  Operator=reciprocal  SignedPower=on  OutDataTypeStr=fixdt(1,32,28)  RndMeth=Zero
  Product : Product
  Switch1 : Switch  Criteria=u2 ~= 0  SaturateOnIntegerOverflow=off  InputSameDT=off
  register : Subsystem
      settings: PortSchema="{\"entries\":[{\"content\":{\"sides\":[{\"content\":{\"connectorIds\":[\"In1\"]},\"type\":\"ConnectorPlacement.EquallySpacedRectSide\",\"uuid\":\"d2805390-6fde-484c-9a7d-6394e985dbe8\"},{\"content\":{\"connectorIds\":[\"Out1\"],\"side\":\"RIGHT\"},\"type\":\"ConnectorPlacement.EquallySpacedRectSide\",\"uuid\":\"b8bae0ca-bbac-4755-ad66-12c0db47e001\"},{\"content\":{\"connectorIds\":[],\"side\":\"TOP\"},\"type\":\"ConnectorPlacement.EquallySpacedRectSide\",\"uuid\":\"3b6f7ac7-ceca-420c-88f8-6d8200a607a4\"},{\"content\":{\"connectorIds\":[\"In2\",\"In3\"],\"side\":\"BOTTOM\"},\"type\":\"ConnectorPlacement.EquallySpacedRectSide\",\"uuid\":\"616043b2-e095-45f8-84b4-1e3ef3d522d8\"}]},\"type\":\"ConnectorPlacement.EquallySpacedConnector\",\"uuid\":\"94d0aeb7-2bda-42be-943a-50da35b391e1\"}],\"packageUris\":[\"http://schema.mathworks.com/mf0/Connector/R2020b\"],\"version\":\"1.0\"}"
  data_out : Outport  VectorParamsAs1DForOutWhenUnconnected=off
  valid_out : Outport  Port=2  OutDataTypeStr=boolean  VectorParamsAs1DForOutWhenUnconnected=off
  wires:
  Delay2/1 -> register/2(valid_in)
  Delay/1 -> Add/1
  Ground/1 -> Switch1/3
  Switch1/1 -> data_out/1
  Logical Operator/1 -> register/3(to_0)
  HDL Counter/2 -> Delay1/1
  HDL Counter/1 -> Math Function/1, Compare To Constant1/1, Compare To Constant/1
  Delay1/1 -> HDL Counter/1
  Compare To Constant/1 -> Logical Operator/1
  Math Function/1 -> Product/2
  valid_in/1 -> Delay2/1, Logical Operator/2, HDL Counter/2
  Add1/1 -> register/1(data_in)  "out"
  Product/1 -> Add1/1
  data_in/1 -> Delay/1
  Add/1 -> Product/1
  Compare To Constant1/1 -> Switch1/2, valid_out/1
  register/1(data_out) -> Goto/1, Add1/2, Add/2
  From/1 -> Switch1/1

== system rx2/demode1/chan_est1/Subsystem/HDL_DUT1/H_est/hRAM1 ==
  H_out : Inport  OutDataTypeStr=fixdt(1,32,27)  PortDimensions=1
  H_valid_out : Inport  Port=2  OutDataTypeStr=boolean
  H_end_out : Inport  Port=3  OutDataTypeStr=boolean
  Compare To Constant : hdlsllib/Logic and Bit Operations/Compare To Constant  relop===  const=10.0  OutDataTypeStr=boolean
  Constant : Constant  OutDataTypeStr=fixdt(0,2,0)
  Constant1 : Constant  OutDataTypeStr=fixdt(0,2,0)
  HDL Counter2 : hdlsllib/Sources/HDL Counter  CountType=Count limited  CountInit=0  CountStep=1  CountMax=11  CountFromType=Initial value  CountFrom=0  CountResetPort=on  CountLoadPort=off  CountEnbPort=on  CountDirPort=off  CountHitOutputPort=off  CountDataType=Unsigned  CountWordLen=8  CountFracLen=0  CountSampTime=1
  Simple Dual Port RAM : hdlsllib/HDL RAMs/Simple Dual Port RAM  ram_size=2
  Out1 : Outport  VectorParamsAs1DForOutWhenUnconnected=off
  wires:
  Compare To Constant/1 -> Simple Dual Port RAM/3
  H_out/1 -> Simple Dual Port RAM/1
  H_valid_out/1 -> HDL Counter2/2
  Constant/1 -> Simple Dual Port RAM/2
  HDL Counter2/1 -> Compare To Constant/1
  Simple Dual Port RAM/1 -> Out1/1
  Constant1/1 -> Simple Dual Port RAM/4
  H_end_out/1 -> HDL Counter2/1

== system rx2/demode1/chan_est1/Subsystem/HDL_DUT1/LS_Est/ctrl_gen ==
  data_in : Inport
  valid_in : Inport  Port=2
  Delay : Delay  DelayLength=1  InitialCondition=0
  Delay1 : Delay  DelayLength=1  InitialCondition=0
  Delay2 : Delay  DelayLength=1  InitialCondition=0
  Detect Fall Nonpositive : hdlsllib/Logic and Bit Operations/Detect Fall Nonpositive  vinit=0  OutDataTypeStr=boolean
  Detect Rise Positive : hdlsllib/Logic and Bit Operations/Detect Rise Positive  vinit=0  OutDataTypeStr=boolean
  Sample Control Bus Creator : whdlutilities/Sample Control Bus Creator
  data_out : Outport
  ctrl_out : Outport  Port=2
  wires:
  Delay2/1 -> data_out/1
  data_in/1 -> Delay2/1
  Delay1/1 -> Detect Rise Positive/1
  Delay/1 -> Sample Control Bus Creator/3
  Sample Control Bus Creator/1 -> ctrl_out/1
  valid_in/1 -> Delay1/1, Detect Fall Nonpositive/1, Delay/1
  Detect Rise Positive/1 -> Sample Control Bus Creator/1
  Detect Fall Nonpositive/1 -> Sample Control Bus Creator/2

== system rx2/demode1/chan_est1/Subsystem/HDL_DUT1/LS_Est/ctrl_gen1 ==
  valid_in : Inport
  Constant : Constant  Value=0
  Data Type Conversion : DataTypeConversion  OutDataTypeStr=boolean  SaturateOnIntegerOverflow=off  RndMeth=Floor
  HDL Counter1 : hdlsllib/Sources/HDL Counter  CountType=Count limited  CountInit=0  CountStep=1  CountMax=1024  CountFromType=Initial value  CountFrom=0  CountResetPort=on  CountLoadPort=off  CountEnbPort=on  CountDirPort=off  CountHitOutputPort=off  CountDataType=Unsigned  CountWordLen=16  CountFracLen=0  CountSampTime=1
  HDL Counter2 : hdlsllib/Sources/HDL Counter  CountType=Count limited  CountInit=0  CountStep=1  CountMax=1  CountFromType=Initial value  CountFrom=0  CountResetPort=off  CountLoadPort=off  CountEnbPort=on  CountDirPort=off  CountHitOutputPort=off  CountDataType=Unsigned  CountWordLen=16  CountFracLen=0  CountSampTime=1
  Logical Operator : Logic  Operator=NOT  AllPortsSameDT=off  OutDataTypeStr=boolean
  Switch : Switch  Threshold=792  OutDataTypeStr=boolean  SaturateOnIntegerOverflow=off  InputSameDT=off
  wvalid_out : Outport  VectorParamsAs1DForOutWhenUnconnected=off
  wires:
  valid_in/1 -> Switch/3, Logical Operator/1, HDL Counter1/2
  Logical Operator/1 -> HDL Counter1/1
  HDL Counter2/1 -> Data Type Conversion/1
  HDL Counter1/1 -> Switch/2
  Constant/1 -> Switch/1
  Switch/1 -> HDL Counter2/1
  Data Type Conversion/1 -> wvalid_out/1

== system rx2/demode1/chan_est1/Subsystem/HDL_DUT1/Pliot/rom ==
  note: rom_pilot = [1+1j;0+0j;-1+1j;0+0j;-1-1j;0+0j;1-1j;0+0j]*1/sqrt(2);
      | rom_pilot_conj = conj(rom_pilot);
      | rom_pilot_conj_tt = fi(rom_pilot_conj,1,16,14);
  note: HDL ROM
  address : Inport
  Direct Lookup Table (n-D) : LookupNDDirect  NumberOfTableDimensions=1  Table=rom_pilot_conj_tt  DiagnosticForOutOfRangeInput=Error
  InputReg : Delay  DelayLength=1
  ResetNoneDelay : Delay  DelayLength=1
  data_out : Outport
  wires:
  ResetNoneDelay/1 -> data_out/1
  address/1 -> InputReg/1
  Direct Lookup Table (n-D)/1 -> ResetNoneDelay/1
  InputReg/1 -> Direct Lookup Table (n-D)/1  "rom_add"

== system rx2/demode1/chan_est1/Subsystem/HDL_DUT1/TA_EST/ctrl_gen ==
  data_in : Inport
      settings: SignalType=complex
  valid_in : Inport  Port=2
  Delay : Delay  DelayLength=1  InitialCondition=0
  Delay1 : Delay  DelayLength=1  InitialCondition=0
  Delay2 : Delay  DelayLength=1  InitialCondition=0
  Detect Fall Nonpositive : hdlsllib/Logic and Bit Operations/Detect Fall Nonpositive  vinit=0  OutDataTypeStr=boolean
  Detect Rise Positive : hdlsllib/Logic and Bit Operations/Detect Rise Positive  vinit=0  OutDataTypeStr=boolean
  Sample Control Bus Creator : whdlutilities/Sample Control Bus Creator
  data_out : Outport
  ctrl_out : Outport  Port=2
  wires:
  Delay2/1 -> data_out/1
  data_in/1 -> Delay2/1
  Delay1/1 -> Detect Rise Positive/1
  Delay/1 -> Sample Control Bus Creator/3
  Sample Control Bus Creator/1 -> ctrl_out/1
  valid_in/1 -> Delay1/1, Detect Fall Nonpositive/1, Delay/1
  Detect Rise Positive/1 -> Sample Control Bus Creator/1
  Detect Fall Nonpositive/1 -> Sample Control Bus Creator/2

== system rx2/demode1/chan_est1/Subsystem/HDL_DUT1/delta_estimator/calculate_norm2 ==
  data_in : Inport
  Complex to Real-Imag2 : ComplexToRealImag
  Dot Product2 : DotProduct  OutDataTypeStr=fixdt(1,64,56)
  Terminator : Terminator
  data_out : Outport
  wires:
  Complex to Real-Imag2/2 -> Terminator/1
  Complex to Real-Imag2/1 -> data_out/1
  data_in/1 -> Dot Product2/1, Dot Product2/2
  Dot Product2/1 -> Complex to Real-Imag2/1

== system rx2/demode1/chan_est1/Subsystem/HDL_DUT1/delta_estimator/calculate_norm3 ==
  data_in : Inport
  Complex to Real-Imag2 : ComplexToRealImag
  Dot Product2 : DotProduct  OutDataTypeStr=fixdt(1,64,56)
  Terminator : Terminator
  data_out : Outport
  wires:
  Dot Product2/1 -> Complex to Real-Imag2/1
  data_in/1 -> Dot Product2/2, Dot Product2/1
  Complex to Real-Imag2/1 -> data_out/1
  Complex to Real-Imag2/2 -> Terminator/1
